simulink model "cic1"  (Simulink 8.1)
settings: Solver=ode45  StartTime=0.0  StopTime=10.0  RelTol=1e-3
values from neighbouring files (symbols this model uses):
  fs_in = 625e6    (= 625000000)    [cic_test.m]    (also in param.m; param2.m)
settings Model: Creator=amr  LastModifiedBy=amr
settings DataIOCC: SignalLoggingSaveFormat=Dataset
settings OptimizationCC: ExpressionDepthLimit=128
settings DebuggingCC: FcnCallInpInsideContextMsg=EnableAllAsError
settings GRTTargetCC: CombineOutputUpdateFcns=on  GRTInterface=off

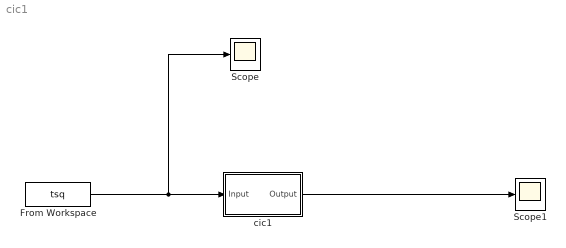
== system cic1 ==
  From Workspace : FromWorkspace  VariableName=tsq  OutDataTypeStr=fixdt(1,16)  SampleTime=1/fs_in  Interpolate=off  OutputAfterFinalValue=Holding final value
  Scope : Scope
  Scope1 : Scope
  cic1 : Subsystem  Tag=FilterWizardSubSystem
      settings: ErrorFcn=dspFilterRealizedInBasicElemsAlgLoopErrFcnCallback
  wires:
  From Workspace/1 -> Scope/1, cic1/1(Input)
  cic1/1(Output) -> Scope1/1

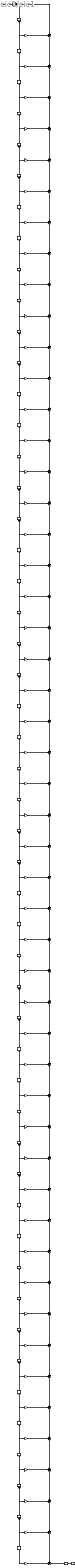
== system cic1/cic1 ==
  Input : Inport
  BodyDelay{2..51} (50 alike) : Delay  DelayLength=1  InitialCondition=0  InputProcessing=Columns as channels (frame based)
  BodyLSum{2..51} (50 alike) : Sum  Inputs=++|  AccumDataTypeStr=fixdt(1,35,32)  OutDataTypeStr=fixdt(1,34,31)  RndMeth=Convergent
  ConvertIn : DataTypeConversion  OutDataTypeStr=fixdt(1,17,16)  RndMeth=Nearest  SaturateOnIntegerOverflow=on
  ConvertOut : DataTypeConversion  OutDataTypeStr=fixdt(1,17,31)  RndMeth=Convergent
  b(1) : Gain  Gain=-0.000919098208468256033  ParamDataTypeStr=fixdt(1,16,16)  OutDataTypeStr=fixdt(1,31,31)  RndMeth=Convergent
  b(10) : Gain  Gain=0.00610545942139436009  ParamDataTypeStr=fixdt(1,16,16)  OutDataTypeStr=fixdt(1,31,31)  RndMeth=Convergent
  b(11) : Gain  Gain=0.0138739157486354008  ParamDataTypeStr=fixdt(1,16,16)  OutDataTypeStr=fixdt(1,31,31)  RndMeth=Convergent
  b(12) : Gain  Gain=0.000350861728290910002  ParamDataTypeStr=fixdt(1,16,16)  OutDataTypeStr=fixdt(1,31,31)  RndMeth=Convergent
  b(13) : Gain  Gain=-0.0169089254366905015  ParamDataTypeStr=fixdt(1,16,16)  OutDataTypeStr=fixdt(1,31,31)  RndMeth=Convergent
  b(14) : Gain  Gain=-0.00890564274915867961  ParamDataTypeStr=fixdt(1,16,16)  OutDataTypeStr=fixdt(1,31,31)  RndMeth=Convergent
  b(15) : Gain  Gain=0.0174411295008548989  ParamDataTypeStr=fixdt(1,16,16)  OutDataTypeStr=fixdt(1,31,31)  RndMeth=Convergent
  b(16) : Gain  Gain=0.0207450445276099009  ParamDataTypeStr=fixdt(1,16,16)  OutDataTypeStr=fixdt(1,31,31)  RndMeth=Convergent
  b(17) : Gain  Gain=-0.0122964942519403  ParamDataTypeStr=fixdt(1,16,16)  OutDataTypeStr=fixdt(1,31,31)  RndMeth=Convergent
  b(18) : Gain  Gain=-0.034240865909578401  ParamDataTypeStr=fixdt(1,16,16)  OutDataTypeStr=fixdt(1,31,31)  RndMeth=Convergent
  b(19) : Gain  Gain=-0.00103452960557239991  ParamDataTypeStr=fixdt(1,16,16)  OutDataTypeStr=fixdt(1,31,31)  RndMeth=Convergent
  b(2) : Gain  Gain=-0.00271769602659550002  ParamDataTypeStr=fixdt(1,16,16)  OutDataTypeStr=fixdt(1,31,31)  RndMeth=Convergent
  b(20) : Gain  Gain=0.0477903055208014974  ParamDataTypeStr=fixdt(1,16,16)  OutDataTypeStr=fixdt(1,31,31)  RndMeth=Convergent
  b(21) : Gain  Gain=0.0273630379148479992  ParamDataTypeStr=fixdt(1,16,16)  OutDataTypeStr=fixdt(1,31,31)  RndMeth=Convergent
  b(22) : Gain  Gain=-0.0593795188310465988  ParamDataTypeStr=fixdt(1,16,16)  OutDataTypeStr=fixdt(1,31,31)  RndMeth=Convergent
  b(23) : Gain  Gain=-0.0823070259292291023  ParamDataTypeStr=fixdt(1,16,16)  OutDataTypeStr=fixdt(1,31,31)  RndMeth=Convergent
  b(24) : Gain  Gain=0.0671869094328705063  ParamDataTypeStr=fixdt(1,16,16)  OutDataTypeStr=fixdt(1,31,31)  RndMeth=Convergent
  b(25) : Gain  Gain=0.310015177090251004  ParamDataTypeStr=fixdt(1,16,16)  OutDataTypeStr=fixdt(1,31,31)  RndMeth=Convergent
  b(26) : Gain  Gain=0.430047880343516986  ParamDataTypeStr=fixdt(1,16,16)  OutDataTypeStr=fixdt(1,31,31)  RndMeth=Convergent
  b(27) : Gain  Gain=0.310015177090251004  ParamDataTypeStr=fixdt(1,16,16)  OutDataTypeStr=fixdt(1,31,31)  RndMeth=Convergent
  b(28) : Gain  Gain=0.0671869094328705063  ParamDataTypeStr=fixdt(1,16,16)  OutDataTypeStr=fixdt(1,31,31)  RndMeth=Convergent
  b(29) : Gain  Gain=-0.0823070259292291023  ParamDataTypeStr=fixdt(1,16,16)  OutDataTypeStr=fixdt(1,31,31)  RndMeth=Convergent
  b(3) : Gain  Gain=-0.00248695275983231009  ParamDataTypeStr=fixdt(1,16,16)  OutDataTypeStr=fixdt(1,31,31)  RndMeth=Convergent
  b(30) : Gain  Gain=-0.0593795188310465988  ParamDataTypeStr=fixdt(1,16,16)  OutDataTypeStr=fixdt(1,31,31)  RndMeth=Convergent
  b(31) : Gain  Gain=0.0273630379148479992  ParamDataTypeStr=fixdt(1,16,16)  OutDataTypeStr=fixdt(1,31,31)  RndMeth=Convergent
  b(32) : Gain  Gain=0.0477903055208014974  ParamDataTypeStr=fixdt(1,16,16)  OutDataTypeStr=fixdt(1,31,31)  RndMeth=Convergent
  b(33) : Gain  Gain=-0.00103452960557239991  ParamDataTypeStr=fixdt(1,16,16)  OutDataTypeStr=fixdt(1,31,31)  RndMeth=Convergent
  b(34) : Gain  Gain=-0.034240865909578401  ParamDataTypeStr=fixdt(1,16,16)  OutDataTypeStr=fixdt(1,31,31)  RndMeth=Convergent
  b(35) : Gain  Gain=-0.0122964942519403  ParamDataTypeStr=fixdt(1,16,16)  OutDataTypeStr=fixdt(1,31,31)  RndMeth=Convergent
  b(36) : Gain  Gain=0.0207450445276099009  ParamDataTypeStr=fixdt(1,16,16)  OutDataTypeStr=fixdt(1,31,31)  RndMeth=Convergent
  b(37) : Gain  Gain=0.0174411295008548989  ParamDataTypeStr=fixdt(1,16,16)  OutDataTypeStr=fixdt(1,31,31)  RndMeth=Convergent
  b(38) : Gain  Gain=-0.00890564274915867961  ParamDataTypeStr=fixdt(1,16,16)  OutDataTypeStr=fixdt(1,31,31)  RndMeth=Convergent
  b(39) : Gain  Gain=-0.0169089254366905015  ParamDataTypeStr=fixdt(1,16,16)  OutDataTypeStr=fixdt(1,31,31)  RndMeth=Convergent
  b(4) : Gain  Gain=0.00366143838350709017  ParamDataTypeStr=fixdt(1,16,16)  OutDataTypeStr=fixdt(1,31,31)  RndMeth=Convergent
  b(40) : Gain  Gain=0.000350861728290910002  ParamDataTypeStr=fixdt(1,16,16)  OutDataTypeStr=fixdt(1,31,31)  RndMeth=Convergent
  b(41) : Gain  Gain=0.0138739157486354008  ParamDataTypeStr=fixdt(1,16,16)  OutDataTypeStr=fixdt(1,31,31)  RndMeth=Convergent
  b(42) : Gain  Gain=0.00610545942139436009  ParamDataTypeStr=fixdt(1,16,16)  OutDataTypeStr=fixdt(1,31,31)  RndMeth=Convergent
  b(43) : Gain  Gain=-0.00769678403706536025  ParamDataTypeStr=fixdt(1,16,16)  OutDataTypeStr=fixdt(1,31,31)  RndMeth=Convergent
  b(44) : Gain  Gain=-0.00655471886964239994  ParamDataTypeStr=fixdt(1,16,16)  OutDataTypeStr=fixdt(1,31,31)  RndMeth=Convergent
  b(45) : Gain  Gain=0.00766530619042168036  ParamDataTypeStr=fixdt(1,16,16)  OutDataTypeStr=fixdt(1,31,31)  RndMeth=Convergent
  b(46) : Gain  Gain=0.0173511659010932989  ParamDataTypeStr=fixdt(1,16,16)  OutDataTypeStr=fixdt(1,31,31)  RndMeth=Convergent
  b(47) : Gain  Gain=0.0136509252306624002  ParamDataTypeStr=fixdt(1,16,16)  OutDataTypeStr=fixdt(1,31,31)  RndMeth=Convergent
  b(48) : Gain  Gain=0.00366143838350709017  ParamDataTypeStr=fixdt(1,16,16)  OutDataTypeStr=fixdt(1,31,31)  RndMeth=Convergent
  b(49) : Gain  Gain=-0.00248695275983231009  ParamDataTypeStr=fixdt(1,16,16)  OutDataTypeStr=fixdt(1,31,31)  RndMeth=Convergent
  b(5) : Gain  Gain=0.0136509252306624002  ParamDataTypeStr=fixdt(1,16,16)  OutDataTypeStr=fixdt(1,31,31)  RndMeth=Convergent
  b(50) : Gain  Gain=-0.00271769602659550002  ParamDataTypeStr=fixdt(1,16,16)  OutDataTypeStr=fixdt(1,31,31)  RndMeth=Convergent
  b(51) : Gain  Gain=-0.000919098208468256033  ParamDataTypeStr=fixdt(1,16,16)  OutDataTypeStr=fixdt(1,31,31)  RndMeth=Convergent
  b(6) : Gain  Gain=0.0173511659010932989  ParamDataTypeStr=fixdt(1,16,16)  OutDataTypeStr=fixdt(1,31,31)  RndMeth=Convergent
  b(7) : Gain  Gain=0.00766530619042168036  ParamDataTypeStr=fixdt(1,16,16)  OutDataTypeStr=fixdt(1,31,31)  RndMeth=Convergent
  b(8) : Gain  Gain=-0.00655471886964239994  ParamDataTypeStr=fixdt(1,16,16)  OutDataTypeStr=fixdt(1,31,31)  RndMeth=Convergent
  b(9) : Gain  Gain=-0.00769678403706536025  ParamDataTypeStr=fixdt(1,16,16)  OutDataTypeStr=fixdt(1,31,31)  RndMeth=Convergent
  Output : Outport
  wires:
  Input/1 -> ConvertIn/1
  b(1)/1 -> BodyLSum2/2
  ConvertIn/1 -> b(1)/1, BodyDelay2/1
  BodyDelay2/1 -> b(2)/1, BodyDelay3/1
  b(2)/1 -> BodyLSum2/1
  BodyLSum2/1 -> BodyLSum3/2
  BodyDelay3/1 -> b(3)/1, BodyDelay4/1
  b(3)/1 -> BodyLSum3/1
  BodyLSum3/1 -> BodyLSum4/2
  BodyDelay4/1 -> b(4)/1, BodyDelay5/1
  b(4)/1 -> BodyLSum4/1
  BodyLSum4/1 -> BodyLSum5/2
  BodyDelay5/1 -> b(5)/1, BodyDelay6/1
  b(5)/1 -> BodyLSum5/1
  BodyLSum5/1 -> BodyLSum6/2
  BodyDelay6/1 -> b(6)/1, BodyDelay7/1
  b(6)/1 -> BodyLSum6/1
  BodyLSum6/1 -> BodyLSum7/2
  BodyDelay7/1 -> b(7)/1, BodyDelay8/1
  b(7)/1 -> BodyLSum7/1
  BodyLSum7/1 -> BodyLSum8/2
  BodyDelay8/1 -> b(8)/1, BodyDelay9/1
  b(8)/1 -> BodyLSum8/1
  BodyLSum8/1 -> BodyLSum9/2
  BodyDelay9/1 -> b(9)/1, BodyDelay10/1
  b(9)/1 -> BodyLSum9/1
  BodyLSum9/1 -> BodyLSum10/2
  BodyDelay10/1 -> b(10)/1, BodyDelay11/1
  b(10)/1 -> BodyLSum10/1
  BodyLSum10/1 -> BodyLSum11/2
  BodyDelay11/1 -> b(11)/1, BodyDelay12/1
  b(11)/1 -> BodyLSum11/1
  BodyLSum11/1 -> BodyLSum12/2
  BodyDelay12/1 -> b(12)/1, BodyDelay13/1
  b(12)/1 -> BodyLSum12/1
  BodyLSum12/1 -> BodyLSum13/2
  BodyDelay13/1 -> b(13)/1, BodyDelay14/1
  b(13)/1 -> BodyLSum13/1
  BodyLSum13/1 -> BodyLSum14/2
  BodyDelay14/1 -> b(14)/1, BodyDelay15/1
  b(14)/1 -> BodyLSum14/1
  BodyLSum14/1 -> BodyLSum15/2
  BodyDelay15/1 -> b(15)/1, BodyDelay16/1
  b(15)/1 -> BodyLSum15/1
  BodyLSum15/1 -> BodyLSum16/2
  BodyDelay16/1 -> b(16)/1, BodyDelay17/1
  b(16)/1 -> BodyLSum16/1
  BodyLSum16/1 -> BodyLSum17/2
  BodyDelay17/1 -> b(17)/1, BodyDelay18/1
  b(17)/1 -> BodyLSum17/1
  BodyLSum17/1 -> BodyLSum18/2
  BodyDelay18/1 -> b(18)/1, BodyDelay19/1
  b(18)/1 -> BodyLSum18/1
  BodyLSum18/1 -> BodyLSum19/2
  BodyDelay19/1 -> b(19)/1, BodyDelay20/1
  b(19)/1 -> BodyLSum19/1
  BodyLSum19/1 -> BodyLSum20/2
  BodyDelay20/1 -> b(20)/1, BodyDelay21/1
  b(20)/1 -> BodyLSum20/1
  BodyLSum20/1 -> BodyLSum21/2
  BodyDelay21/1 -> b(21)/1, BodyDelay22/1
  b(21)/1 -> BodyLSum21/1
  BodyLSum21/1 -> BodyLSum22/2
  BodyDelay22/1 -> b(22)/1, BodyDelay23/1
  b(22)/1 -> BodyLSum22/1
  BodyLSum22/1 -> BodyLSum23/2
  BodyDelay23/1 -> b(23)/1, BodyDelay24/1
  b(23)/1 -> BodyLSum23/1
  BodyLSum23/1 -> BodyLSum24/2
  BodyDelay24/1 -> b(24)/1, BodyDelay25/1
  b(24)/1 -> BodyLSum24/1
  BodyLSum24/1 -> BodyLSum25/2
  BodyDelay25/1 -> b(25)/1, BodyDelay26/1
  b(25)/1 -> BodyLSum25/1
  BodyLSum25/1 -> BodyLSum26/2
  BodyDelay26/1 -> b(26)/1, BodyDelay27/1
  b(26)/1 -> BodyLSum26/1
  BodyLSum26/1 -> BodyLSum27/2
  BodyDelay27/1 -> b(27)/1, BodyDelay28/1
  b(27)/1 -> BodyLSum27/1
  BodyLSum27/1 -> BodyLSum28/2
  BodyDelay28/1 -> b(28)/1, BodyDelay29/1
  b(28)/1 -> BodyLSum28/1
  BodyLSum28/1 -> BodyLSum29/2
  BodyDelay29/1 -> b(29)/1, BodyDelay30/1
  b(29)/1 -> BodyLSum29/1
  BodyLSum29/1 -> BodyLSum30/2
  BodyDelay30/1 -> b(30)/1, BodyDelay31/1
  b(30)/1 -> BodyLSum30/1
  BodyLSum30/1 -> BodyLSum31/2
  BodyDelay31/1 -> b(31)/1, BodyDelay32/1
  b(31)/1 -> BodyLSum31/1
  BodyLSum31/1 -> BodyLSum32/2
  BodyDelay32/1 -> b(32)/1, BodyDelay33/1
  b(32)/1 -> BodyLSum32/1
  BodyLSum32/1 -> BodyLSum33/2
  BodyDelay33/1 -> b(33)/1, BodyDelay34/1
  b(33)/1 -> BodyLSum33/1
  BodyLSum33/1 -> BodyLSum34/2
  BodyDelay34/1 -> b(34)/1, BodyDelay35/1
  b(34)/1 -> BodyLSum34/1
  BodyLSum34/1 -> BodyLSum35/2
  BodyDelay35/1 -> b(35)/1, BodyDelay36/1
  b(35)/1 -> BodyLSum35/1
  BodyLSum35/1 -> BodyLSum36/2
  BodyDelay36/1 -> b(36)/1, BodyDelay37/1
  b(36)/1 -> BodyLSum36/1
  BodyLSum36/1 -> BodyLSum37/2
  BodyDelay37/1 -> b(37)/1, BodyDelay38/1
  b(37)/1 -> BodyLSum37/1
  BodyLSum37/1 -> BodyLSum38/2
  BodyDelay38/1 -> b(38)/1, BodyDelay39/1
  b(38)/1 -> BodyLSum38/1
  BodyLSum38/1 -> BodyLSum39/2
  BodyDelay39/1 -> b(39)/1, BodyDelay40/1
  b(39)/1 -> BodyLSum39/1
  BodyLSum39/1 -> BodyLSum40/2
  BodyDelay40/1 -> b(40)/1, BodyDelay41/1
  b(40)/1 -> BodyLSum40/1
  BodyLSum40/1 -> BodyLSum41/2
  BodyDelay41/1 -> b(41)/1, BodyDelay42/1
  b(41)/1 -> BodyLSum41/1
  BodyLSum41/1 -> BodyLSum42/2
  BodyDelay42/1 -> b(42)/1, BodyDelay43/1
  b(42)/1 -> BodyLSum42/1
  BodyLSum42/1 -> BodyLSum43/2
  BodyDelay43/1 -> b(43)/1, BodyDelay44/1
  b(43)/1 -> BodyLSum43/1
  BodyLSum43/1 -> BodyLSum44/2
  BodyDelay44/1 -> b(44)/1, BodyDelay45/1
  b(44)/1 -> BodyLSum44/1
  BodyLSum44/1 -> BodyLSum45/2
  BodyDelay45/1 -> b(45)/1, BodyDelay46/1
  b(45)/1 -> BodyLSum45/1
  BodyLSum45/1 -> BodyLSum46/2
  BodyDelay46/1 -> b(46)/1, BodyDelay47/1
  b(46)/1 -> BodyLSum46/1
  BodyLSum46/1 -> BodyLSum47/2
  BodyDelay47/1 -> b(47)/1, BodyDelay48/1
  b(47)/1 -> BodyLSum47/1
  BodyLSum47/1 -> BodyLSum48/2
  BodyDelay48/1 -> b(48)/1, BodyDelay49/1
  b(48)/1 -> BodyLSum48/1
  BodyLSum48/1 -> BodyLSum49/2
  BodyDelay49/1 -> b(49)/1, BodyDelay50/1
  b(49)/1 -> BodyLSum49/1
  BodyLSum49/1 -> BodyLSum50/2
  BodyDelay50/1 -> b(50)/1, BodyDelay51/1
  b(50)/1 -> BodyLSum50/1
  BodyLSum50/1 -> BodyLSum51/1
  BodyDelay51/1 -> b(51)/1
  b(51)/1 -> BodyLSum51/2
  BodyLSum51/1 -> ConvertOut/1
  ConvertOut/1 -> Output/1
